simulink model "two_virtual_wheel_analog"  (Simulink 7.8)
settings: Solver=ode3  StartTime=0.0  StopTime=tfinal  FixedStep=Deltat  RelTol=1e-3
undefined symbols (not defined in the file): Jw1, Jw2, k1, k2, step_time, Theta_z_0
settings Model: Creator=Embed_Sys_course  LastModifiedBy=Embed_Sys_course  ExtModeTrigMode=oneshot  ExtModeArmWhenConnect=off
settings DataIOCC: LimitDataPoints=off
settings OptimizationCC: BooleanDataType=off  InitFltsAndDblsToZero=on
settings DebuggingCC: SaveWithParameterizedLinksMsg=none  SignalResolutionControl=TryResolveAllWithWarning  SolverPrmCheckMsg=none  MultiTaskDSMMsg=warning  MultiTaskCondExecSysMsg=none  StrictBusMsg=None
settings HardwareCC: TargetUnknown=on
settings RTWCC: IncludeERTFirstTime=on
settings CodeAppCC: CustomSymbolStrType=$N$R$M_T
settings GRTTargetCC: TargetFcnLib=ansi_tfl_tmw.mat  TargetFunctionLibrary=NOT IN USE  CPPClassGenCompliant=on

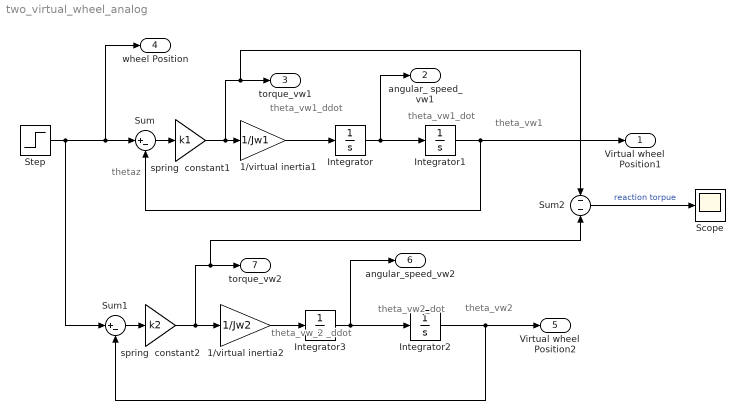
== system two_virtual_wheel_analog ==
  note: theta_vw1
  note: theta_vw1_dot
  note: theta_vw1_ddot
  note: thetaz
  note: theta_vw2
  note: theta_vw2_dot
  note: theta_vw_2
      | _ddot
  1/virtual inertia1 : Gain  Gain=1/Jw1  SaturateOnIntegerOverflow=on  OutDataTypeStr=Inherit: Same as input  ParamDataTypeStr=Inherit: Same as input
  1/virtual inertia2 : Gain  Gain=1/Jw2  SaturateOnIntegerOverflow=on  OutDataTypeStr=Inherit: Same as input  ParamDataTypeStr=Inherit: Same as input
  Integrator{,1..3} (4 alike) : Integrator
  Scope : Scope
  Step : Step  Time=step_time  After=Theta_z_0  SampleTime=0
  Sum : Sum  Inputs=|+-  SaturateOnIntegerOverflow=on  InputSameDT=on  OutDataTypeStr=Inherit: Same as first input
  Sum1 : Sum  Inputs=|+-  SaturateOnIntegerOverflow=on  InputSameDT=on  OutDataTypeStr=Inherit: Same as first input
  Sum2 : Sum  Inputs=-|-  SaturateOnIntegerOverflow=on  InputSameDT=on  OutDataTypeStr=Inherit: Same as first input
  spring  constant1 : Gain  Gain=k1  SaturateOnIntegerOverflow=on  OutDataTypeStr=Inherit: Same as input  ParamDataTypeStr=Inherit: Same as input
  spring  constant2 : Gain  Gain=k2  SaturateOnIntegerOverflow=on  OutDataTypeStr=Inherit: Same as input  ParamDataTypeStr=Inherit: Same as input
  Virtual wheel     Position1 : Outport
  angular_ speed_ vw1 : Outport  Port=2
  torque_vw1 : Outport  Port=3
  wheel Position : Outport  Port=4
  Virtual wheel     Position2 : Outport  Port=5
  angular_speed_vw2 : Outport  Port=6
  torque_vw2 : Outport  Port=7
  wires:
  Integrator1/1 -> Virtual wheel     Position1/1, Sum/2
  Sum/1 -> spring  constant1/1
  Step/1 -> wheel Position/1, Sum/1, Sum1/1
  spring  constant1/1 -> 1/virtual inertia1/1, torque_vw1/1, Sum2/1
  1/virtual inertia1/1 -> Integrator/1
  Integrator/1 -> angular_ speed_ vw1/1, Integrator1/1
  Integrator2/1 -> Sum1/2, Virtual wheel     Position2/1
  Sum1/1 -> spring  constant2/1
  spring  constant2/1 -> 1/virtual inertia2/1, torque_vw2/1, Sum2/2
  1/virtual inertia2/1 -> Integrator3/1
  Integrator3/1 -> angular_speed_vw2/1, Integrator2/1
  Sum2/1 -> Scope/1  "reaction torpue"
